simulink model "dynamicModelQuaternions"  (R2015b)
settings: Solver=FixedStepAuto  StartTime=0.0  StopTime=inf  FixedStep=1/60  RelTol=1e-3
undefined symbols (not defined in the file or in its folder): Earth, WGS84
libraries: aerolibfltsims x3, aerolibconvert2 x2, aerolibanimutils x2, aerolibtransform2 x1
settings Model: Creator=fidel  LastModifiedBy=fidel

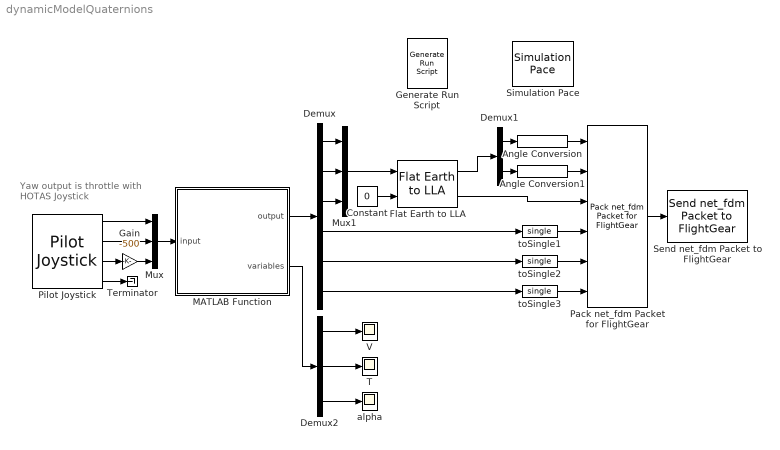
== system dynamicModelQuaternions ==
  note: Yaw output is throttle
      | with HOTAS Joystick
  Angle Conversion : aerolibconvert2/Angle Conversion  IU=deg  OU=rad
  Angle Conversion1 : aerolibconvert2/Angle Conversion  IU=deg  OU=rad
  Constant : Constant  Value=0
  Demux : Demux  Outputs=6
  Demux1 : Demux  Outputs=2
  Demux2 : Demux  Outputs=3
  Flat Earth to LLA : aerolibtransform2/Flat Earth to LLA  units=Metric (MKS)  ptype=Earth (WGS84)  F=1/298.257223563  R=6378137  LL0=[0 10]  psi=90
  Gain : Gain  Gain=-500
  Generate Run Script : aerolibfltsims/Generate Run Script  OutputFileName=optimFP_runFG.bat  FlightGearBaseDirectory=C:\Program Files\FlightGear 2016.4.4  GeometryModelName=ZivkoEdge540  DestinationPort=5502  OriginAddress=127.0.0.1  OriginPort=5505  LocalAddress=127.0.0.1  AirportId=KSFO  RunwayId=10L  InitialAltitude=7224  InitialHeading=113  OffsetDistance=4.72  OffsetAzimuth=0  GenerateFile=off  Architecture=Default  dataFlow=Send
  MATLAB Function : MATLAB Function  TreatAsAtomicUnit=on
  Mux : Mux  Inputs=3
  Mux1 : Mux  Inputs=3
  Pack net_fdm Packet for FlightGear : aerolibfltsims/Pack net_fdm Packet for FlightGear  FlightGearVersion=v3.4  ShowPositionAttitudeInputs=on  ShowVelocityAccelerationInputs=off  ShowControlSurfacePositionInputs=off  ShowEngineFuelInputs=off  ShowLandingGearInputs=off  ShowEnvironmentInputs=off  SampleTime=-1
  Pilot Joystick : aerolibanimutils/Pilot Joystick  JoystickID=Joystick1  OutputConfiguration=FourAxis  SampleTime=1/60
  Send net_fdm Packet to FlightGear : aerolibfltsims/Send net_fdm Packet to FlightGear  DestinationIpAddress=127.0.0.1  DestinationPort=5502  LocalIpPort=-1  varLen=off  SampleTime=-1
  Simulation Pace : aerolibanimutils/Simulation Pace  SimulationPace=1  SleepMode=MATLAB Thread  OutputPaceError=off  SampleTime=-1
      settings: AttributesFormatString=%<SimulationPace> sec/sec
  T : Scope
  Terminator : Terminator
  V : Scope
  alpha : Scope
  toSingle1 : DataTypeConversion  OutDataTypeStr=single
  toSingle2 : DataTypeConversion  OutDataTypeStr=single
  toSingle3 : DataTypeConversion  OutDataTypeStr=single
  wires:
  Angle Conversion1/1 -> Pack net_fdm Packet for FlightGear/2
  Angle Conversion/1 -> Pack net_fdm Packet for FlightGear/1
  toSingle3/1 -> Pack net_fdm Packet for FlightGear/6
  toSingle2/1 -> Pack net_fdm Packet for FlightGear/5
  toSingle1/1 -> Pack net_fdm Packet for FlightGear/4
  Pack net_fdm Packet for FlightGear/1 -> Send net_fdm Packet to FlightGear/1
  Demux/6 -> toSingle3/1
  Demux/1 -> Mux1/1
  Demux/2 -> Mux1/2
  Demux/3 -> Mux1/3
  Demux/4 -> toSingle1/1
  Demux/5 -> toSingle2/1
  Pilot Joystick/3 -> Gain/1
  Pilot Joystick/1 -> Mux/1
  Pilot Joystick/2 -> Mux/2
  Pilot Joystick/4 -> Terminator/1
  Mux/1 -> MATLAB Function/1(input)
  MATLAB Function/1(output) -> Demux/1
  Flat Earth to LLA/1 -> Demux1/1
  Flat Earth to LLA/2 -> Pack net_fdm Packet for FlightGear/3
  Mux1/1 -> Flat Earth to LLA/1
  Demux1/1 -> Angle Conversion/1
  Demux1/2 -> Angle Conversion1/1
  Constant/1 -> Flat Earth to LLA/2
  MATLAB Function/2(variables) -> Demux2/1
  Demux2/1 -> V/1
  Demux2/2 -> T/1
  Demux2/3 -> alpha/1
  Gain/1 -> Mux/3

== matlab function dynamicModelQuaternions/MATLAB Function ==
  data: input input; output output; variables output
function [output,variables] = fcn(input)

    p = input(1);
    alpha_dot = input(2);
    T_dot = input(3);
    
    persistent T;
    persistent V;
    persistent alpha;
    persistent q0;
    persistent q1;
    persistent q2;
    persistent q3;
    persistent x;
    persistent y;
    persistent h;
    
    persistent Tmax;
    persistent Tmin;
    persistent m;
    persistent g;
    persistent rho;
    persistent S;
    persistent Clalpha;
    persistent K;
    persistent Cd0;
    persistent alpha_min;
    persistent alpha_max;

    persistent roll;
    persistent pitch;
    persistent yaw;
    persistent dt;
    
    if isempty(T)
        T = 5000;
        V = 90;
        alpha = 0.1;
        q0 = 1;
        q1 = 0;
        q2 = 0;
        q3 = 0;
        x = 0;
        y = 0;
        h = 1500;
        Tmax = 9000;
        Tmin = 0;
        m = 750;
        g = 9.81;
        rho = 1.225;
        S = 9.1;
        Clalpha = 1.3;
        K = 0.1779;
        Cd0 = 0.036;
        alpha_min = -0.5;
        alpha_max = 0.5;
        dt = 1/60;
    end
    
    T = max(min(T + T_dot*dt, Tmax), Tmin);
    alpha = max(min(alpha + alpha_dot*dt, alpha_max), alpha_min);
    Cl = Clalpha*alpha;
    L = 0.5*rho*V^2*S*Cl;
    D = 0.5*rho*V^2*S*(Cd0+K*Cl^2);
    q = (T*sin(alpha)+L-m*g*(q0^2-q1^2-q2^2+q3^2))/(m*V);
    r = (2*m*g*(q0*q1+q2*q3))/(m*V);
    V_dot = (T*cos(alpha)-D+2*m*g*(q1*q3-q0*q2))/m;
    q0_dot = -0.5*(q1*p+q2*q+q3*r);
    q1_dot =  0.5*(q0*p+q2*r-q3*q);
    q2_dot =  0.5*(q0*q+q3*p-q1*r);
    q3_dot =  0.5*(q0*r+q1*q-q2*p);
    V = V + V_dot*dt;
    q0 = q0 + q0_dot*dt;
    q1 = q1 + q1_dot*dt;
    q2 = q2 + q2_dot*dt;
    q3 = q3 + q3_dot*dt;
    qnorm = sqrt(q0^2+q1^2+q2^2+q3^2);
    q0 = q0 / qnorm;
    q1 = q1 / qnorm;
    q2 = q2 / qnorm;
    q3 = q3 / qnorm;
    x_dot = V*(q0^2+q1^2-q2^2-q3^2);
    y_dot = 2*V*(q0*q3+q1*q2);
    h_dot = 2*V*(q0*q2-q1*q3);
    x = x + x_dot*dt;
    y = y + y_dot*dt;
    h = h + h_dot*dt;
    [euler] = quat2eul([q0 q1 q2 q3],'ZYX');
    yaw = euler(1);
    pitch = euler(2);
    roll = euler(3);

    output = [x;-y;-h;roll;pitch;yaw];
    variables = [V;T;alpha];
